simulink model "smcSL_implementacion"  (R2022b)
settings: Solver=FixedStepAuto  StartTime=0.0  StopTime=inf  EnableMultiTasking=on
values from neighbouring files (symbols this model uses):
  a = 1    [SMC.mat]
  beta = 40    [SMC.mat]
undefined symbols (not defined in the file or in its folder): A, B, C, d1, d2, delta, I, L, miu, wb, wcp, wm
libraries: arduinolib x2, simulink x1
settings Model: ExtModeTrigDuration=2  Creator=andre  LastModifiedBy=amoralesma
settings SolverCC: ZeroCrossAlgorithm=Adaptive  AlgebraicLoopSolver=TrustRegion
settings OptimizationCC: EnhancedBackFolding=on  PassReuseOutputArgsAs=Individual arguments  ZeroExternalMemoryAtStartup=off  ZeroInternalMemoryAtStartup=off  MaxStackSize=64  OptimizeBlockOrder=speed  DifferentSizesBufferReuse=on  OptimizationCustomize=off  EfficientTunableParamExpr=on
settings DebuggingCC: IgnoredZcDiagnostic=none  ParameterTunabilityLossMsg=error  UnconnectedInputMsg=warning  UnconnectedOutputMsg=warning  UnconnectedLineMsg=warning  SFMachineParentedDataDiag=warning
settings HardwareCC: ProdBitPerInt=16  ProdBitPerPointer=16  ProdBitPerSizeT=16  ProdBitPerPtrDiffT=16  ProdLargestAtomicFloat=None  ProdWordSize=8  ProdHWDeviceType=Atmel->AVR  UseEmbeddedCoderFeatures=off  UseSimulinkCoderFeatures=off
settings ModelReferenceCC: EnableRefExpFcnMdlSchedulingChecks=on
settings SFSimCC: MATLABDynamicMemAlloc=off
settings RTWCC: Description=Embedded Coder  SystemTargetFile=ert.tlc  HardwareBoard=Arduino Uno  TLCOptions=-aInlineSetEventsForThisBaseRateFcn=TLC_FALSE -aSuppressMultiTaskScheduler=TLC_FALSE -aRateBasedStepFcn=1  TemplateMakefile=ert_default_tmf  Toolchain=Arduino AVR  BuildConfiguration=Faster Runs  DLArmComputeVersion=19.05
settings CodeAppCC: ForceParamTrailComments=on  IgnoreCustomStorageClasses=off  OperatorAnnotations=on  SimulinkDataObjDesc=on  SFDataObjDesc=on  InsertBlockDesc=on
settings ERTTargetCC: SupportContinuousTime=on  SupportNonInlinedSFcns=on  SupportVariableSizeSignals=on  ExtModeTransport=3  ExtModeStaticAlloc=on  ExtModeAutomaticAllocSize=off  ExtModeStaticAllocSize=250  ExtModeMexFile=ext_xcp  ExtModeIntrfLevel=Level2 - Open

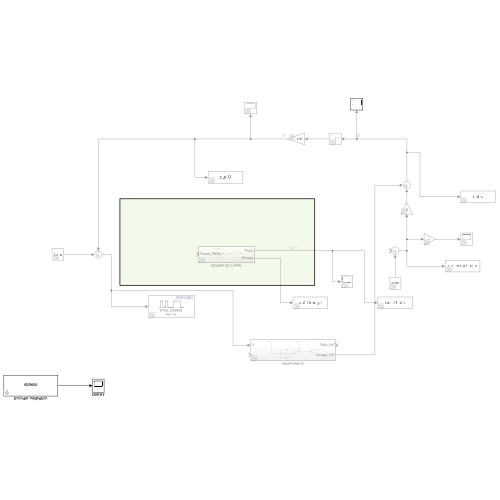
[thumbnail: Simulink's stored preview of the top-level diagram]
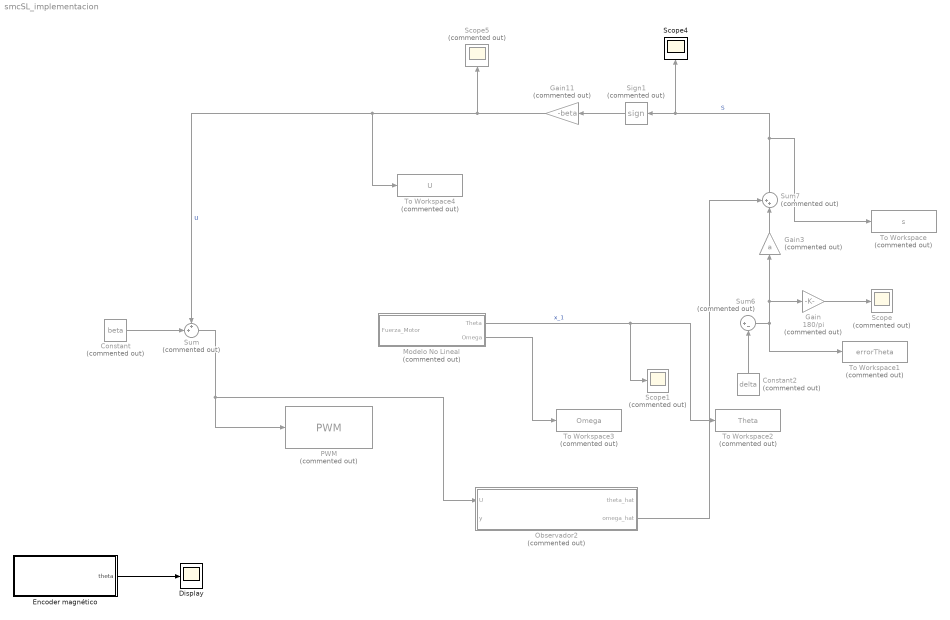
== system smcSL_implementacion ==
  Constant : Constant  Commented=on  Value=beta
  Constant2 : Constant  Commented=on  Value=delta
  Display : Scope
  Encoder magnético : Subsystem
      mask Display: disp('AS5600');
  Gain : Gain  Commented=on  Gain=180/pi
  Gain11 : Gain  Commented=on  Gain=-beta
  Gain3 : Gain  Commented=on  Gain=a
  Modelo No Lineal : Subsystem  Commented=on
  Observador2 : Subsystem  Commented=on
  PWM : arduinolib/PWM  Commented=on  pinNumber=9  frequencyType=Default  desiredFrequency=490.2  achievableFrequency=490.2
  Scope : Scope  Commented=on
  Scope1 : Scope  Commented=on
  Scope4 : Scope
  Scope5 : Scope  Commented=on
  Sign1 : Signum  Commented=on  ZeroCross=off
  Sum : Sum  Commented=on  Inputs=++|
  Sum6 : Sum  Commented=on  Inputs=|+-
  Sum7 : Sum  Commented=on  Inputs=++|
  To Workspace : ToWorkspace  Commented=on  VariableName=s  SaveFormat=Timeseries  SampleTime=-1
  To Workspace1 : ToWorkspace  Commented=on  VariableName=errorTheta  SaveFormat=Timeseries  SampleTime=-1
  To Workspace2 : ToWorkspace  Commented=on  VariableName=Theta  SaveFormat=Timeseries  SampleTime=-1
  To Workspace3 : ToWorkspace  Commented=on  VariableName=Omega  SaveFormat=Timeseries  SampleTime=-1
  To Workspace4 : ToWorkspace  Commented=on  VariableName=U  SaveFormat=Timeseries  SampleTime=-1
  wires:
  Sign1/1 -> Gain11/1
  Gain3/1 -> Sum7/2
  Sum6/1 -> Gain/1, Gain3/1, To Workspace1/1
  Modelo No Lineal/1(Theta) -> Scope1/1, To Workspace2/1  "x_1"
  Sum7/1 -> To Workspace/1, Scope4/1, Sign1/1  "S"
  Gain11/1 -> To Workspace4/1, Sum/1, Scope5/1  "U"
  Constant2/1 -> Sum6/2
  Modelo No Lineal/2(Omega) -> To Workspace3/1
  Constant/1 -> Sum/2
  Sum/1 -> Observador2/1(U), PWM/1
  Gain/1 -> Scope/1
  Observador2/2(omega_hat) -> Sum7/1
  Encoder magnético/1(theta) -> Display/1

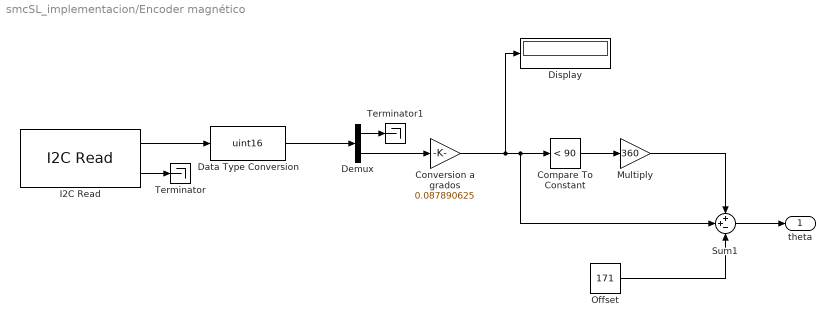
== system smcSL_implementacion/Encoder magnético ==
  Compare To Constant : simulink/Logic and Bit Operations/Compare To Constant  relop=<  const=90  OutDataTypeStr=uint8
  Conversion a grados : Gain  Gain=0.087890625
  Data Type Conversion : DataTypeConversion  OutDataTypeStr=uint16  SaturateOnIntegerOverflow=off  RndMeth=Floor
  Demux : Demux  Outputs=2
  Display : Display
  I2C Read : arduinolib/I2C Read  I2CModule=0  Mode=Master  SlaveAddress=0x36  SlaveByteOrder=BigEndian  Direction=Receiver  RegisterAddressMode=on  RegisterAddress=0x0C  SlaveDataType=uint16  DataLength=2  NoAck=off  RepeatedStart=off  OutputStatus=on  blockPlatform=ARDUINO  SampleTime=0.003
  Multiply : Gain  Gain=360
  Offset : Constant  Value=171
  Sum1 : Sum  Inputs=++-
  Terminator : Terminator
  Terminator1 : Terminator
  theta : Outport
  wires:
  Demux/2 -> Conversion a grados/1
  Data Type Conversion/1 -> Demux/1
  Offset/1 -> Sum1/3
  I2C Read/1 -> Data Type Conversion/1
  Multiply/1 -> Sum1/1
  Conversion a grados/1 -> Display/1, Compare To Constant/1, Sum1/2
  Compare To Constant/1 -> Multiply/1
  I2C Read/2 -> Terminator/1
  Sum1/1 -> theta/1
  Demux/1 -> Terminator1/1

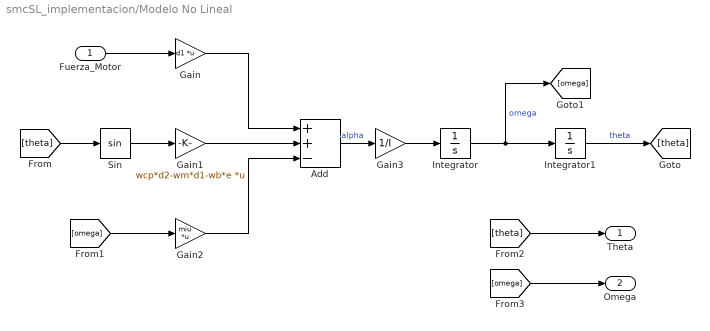
== system smcSL_implementacion/Modelo No Lineal ==
  Fuerza_Motor : Inport
  Add : Sum  Inputs=++-
  Gain : Gain  Gain=d1  Multiplication=Matrix(K*u)
  Gain1 : Gain  Gain=wcp*d2-wm*d1-wb*e  Multiplication=Matrix(K*u)
  Gain2 : Gain  Gain=miu  Multiplication=Matrix(K*u)
  Gain3 : Gain  Gain=1/I
  Integrator : Integrator  ZeroCross=off
  Integrator1 : Integrator  InitialCondition=pi/2  ZeroCross=off
  Sin : Trigonometry  ApproximationMethod=CORDIC
  Theta : Outport
  Omega : Outport  Port=2
  wires:
  [omega] -> Omega/1
  Gain1/1 -> Add/2
  Integrator/1 -> [omega], Integrator1/1  "omega"
  Fuerza_Motor/1 -> Gain/1
  Integrator1/1 -> [theta]  "theta"
  Gain2/1 -> Add/3
  Gain/1 -> Add/1
  Add/1 -> Gain3/1  "alpha"
  [theta] -> Sin/1
  [omega] -> Gain2/1
  [theta] -> Theta/1
  Sin/1 -> Gain1/1
  Gain3/1 -> Integrator/1

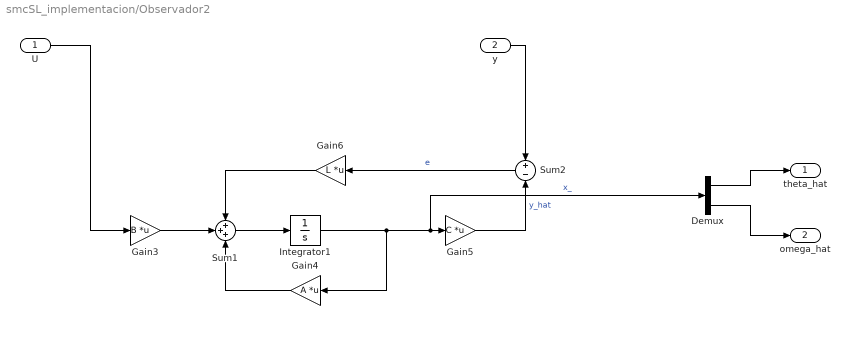
== system smcSL_implementacion/Observador2 ==
  U : Inport
  y : Inport  Port=2
  Demux : Demux  Outputs=2
  Gain3 : Gain  Gain=B  Multiplication=Matrix(K*u)
  Gain4 : Gain  Gain=A  Multiplication=Matrix(K*u)
  Gain5 : Gain  Gain=C  Multiplication=Matrix(K*u)
  Gain6 : Gain  Gain=L  Multiplication=Matrix(K*u)
  Integrator1 : Integrator  InitialCondition=[deg2rad(10), 0]
  Sum1 : Sum  Inputs=+++
  Sum2 : Sum  Inputs=+|-
  theta_hat : Outport
  omega_hat : Outport  Port=2
  wires:
  U/1 -> Gain3/1
  y/1 -> Sum2/1
  Gain5/1 -> Sum2/2  "y_hat"
  Sum1/1 -> Integrator1/1
  Gain3/1 -> Sum1/2
  Gain6/1 -> Sum1/1
  Integrator1/1 -> Gain4/1, Demux/1, Gain5/1  "x_"
  Sum2/1 -> Gain6/1  "e"
  Gain4/1 -> Sum1/3
  Demux/1 -> theta_hat/1
  Demux/2 -> omega_hat/1
